simulink model "w2p3"  (R2020b)
settings: Solver=VariableStepAuto  StartTime=0.0  StopTime=120  RelTol=1e-3
model workspace (MAT data in the model file):
  Kd = Simulink.Parameter
  Kd.Value = 484.0516
  Kd.DataType = 'auto'
  Kd.Dimensions = [1 1]
  Ki = Simulink.Parameter
  Ki.Value = 350
  Ki.DataType = 'auto'
  Ki.Dimensions = [1 1]
  Kp = Simulink.Parameter
  Kp.Value = 495.0505
  Kp.DataType = 'auto'
  Kp.Dimensions = [1 1]
  b = Simulink.Parameter
  b.Value = 50
  b.DataType = 'auto'
  b.Dimensions = [1 1]
  m = Simulink.Parameter
  m.Value = 1000
  m.DataType = 'auto'
  m.Dimensions = [1 1]
settings Model: Creator=Dell  LastModifiedBy=Dell

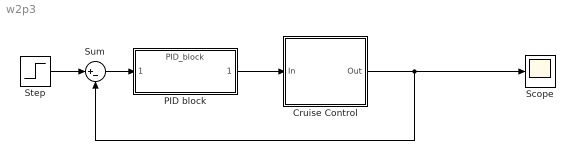
== system w2p3 ==
  Cruise Control : Subsystem
  PID block : ModelReference  ModelNameDialog=PID_block  SimulationMode=Normal  ModelReferenceVersion=1.9
  Scope : Scope
  Step : Step  Time=0  After=500  SampleTime=0
  Sum : Sum  Inputs=|+-
  wires:
  Cruise Control/1(Out) -> Scope/1, Sum/2
  PID block/1 -> Cruise Control/1(In)
  Step/1 -> Sum/1
  Sum/1 -> PID block/1

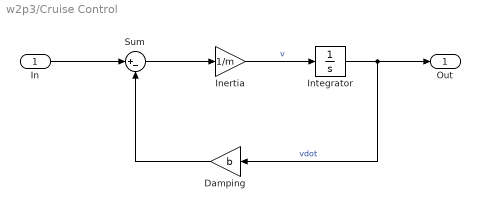
== system w2p3/Cruise Control ==
  In : Inport
  Damping : Gain  Gain=b
  Inertia : Gain  Gain=1/m
  Integrator : Integrator
  Sum : Sum  Inputs=|+-
  Out : Outport
  wires:
  Inertia/1 -> Integrator/1  "v"
  Sum/1 -> Inertia/1
  Integrator/1 -> Out/1, Damping/1  "vdot"
  Damping/1 -> Sum/2
  In/1 -> Sum/1
